simulink model "Battery_droop_control_4"  (R2022a)
settings: Solver=ode23tb  StartTime=0.0  StopTime=1  RelTol=1e-3  EnableMultiTasking=on
values from neighbouring files (symbols this model uses):
  R_power_mode_load_change = zeros(1, length(load_percent_list))    [Battery_charge_discharge_FSBB_param_init.m]
  R_voltage_mode_load_change = zeros(1, length(load_percent_list))    [Battery_charge_discharge_FSBB_param_init.m]
  time_step = 1 / wave_freq    (= 2.22222222222e-05)    [Battery_charge_discharge_FSBB_param_init.m]
undefined symbols (not defined in the file or in its folder): Ion, Lithium
libraries: spsSeriesRLCBranchLib x27, spsTriangleGeneratorLib x16, slpidlib x14, spsCurrentMeasurementLib x9, spsIGBTDiodeLib x8, spsIdealSwitchLib x8, spsVoltageMeasurementLib x8, simulink x4, spsBatteryLib x3, spsControlledVoltageSourceLib x3, eeGeneralControl x2, spspowerguiLib x1
(part 2 of 4)

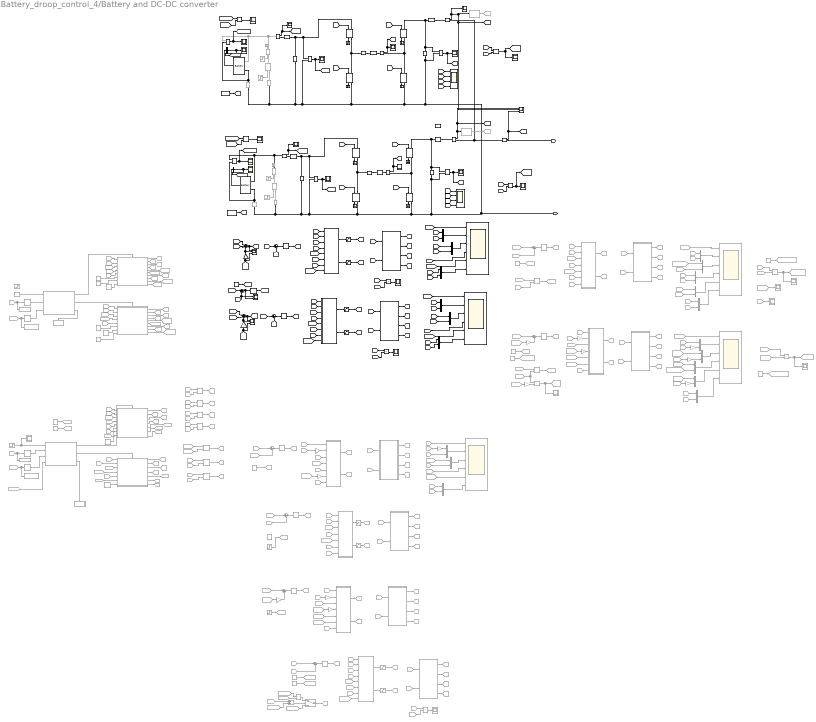
== system Battery_droop_control_4/Battery and DC-DC converter ==
  note: Discharge in Constant Power Mode : realize by constant current
  note: Be charged in constant Current Mode
  note: Discharge in constant Current Mode
  note: Discharge in constant Voltage Mode
  note: FSBB Passivity Based Control
      | control algorithm ref: https://www.youtube.com/watch?v=5YT7cERlMrg
      | 1. Modify the topology corresponding to Gosspower hardware.
      | 1.1 add additional capacities in both input and output side
      | 1.2 add additional 2.2e-6H inductor in both input and output side to mitigate the fluctuation in constant current mode.
      | 2. Realize the constant current/voltage/Power mode in charge/discharge mode.
      |
      | Author LokiXun rongji.xun@gmail.com
  note: Be Charged in constant Voltage Mode
  note: Be Charged in Constant Power Mode : realize by constant current
  note: Constant Current/Power Transition Point
  note: Charge Mode Transition
  note: Discharge Mode Transition
  note: Discharge in Constant Current Mode using Voltage control
  note: Charge Mode
  note: Discharge Mode
  note: I_imax = 31.25A; Ubus_min = 95.5V; Ubus_ref = 96V;
  note: I_imax = 31.25A; Ubus_min = 95.5V; Ubus_ref = 96V;
  note: 和开关频率同步
  note: Discharge in constant Voltage Mode
  note: 和开关频率同步
  "85 volts, 100 Ah LithiumIon battery " : spsBatteryLib/Battery  BatType=Lithium-Ion  ShowTempParam=off  ThermalPreset=no  ShowAgeParam=off  NomV=85  NomQ=100  SOC=20  Batt_Tr=30  PresetModel=off  MaxQ=107.6923  MinV=83.2  FullV=115.2  Dis_rate=43.4783  R=0.08  Normal_OP=96.1538  expZone=[92.2034, 20]  current=[6.5 13 32.5]  Units=Time  Tci=20  NomT=20  T2=-30  MaxQ2=4.8  FullV2=7.1  Normal_OP2=5.655  expZone2="[6.58           1]"  Rca=0.6  ti=2000  Dp=0  Neq0=0  Tsim=1e6  Ta1=25  Qeol=5.4*0.9  Reol=0.013333*1.2  Char_age=[2.3478, 3]  Dis_age=[2.3478, 10]  N1=1500  N2=10500  N3=1000  N4=1400  Ta2=45  N5=950
  "85 volts, 100 Ah LithiumIon battery 2" : spsBatteryLib/Battery  BatType=Lithium-Ion  ShowTempParam=off  ThermalPreset=no  ShowAgeParam=off  NomV=85  NomQ=100  SOC=20  Batt_Tr=30  PresetModel=off  MaxQ=107.6923  MinV=83.2  FullV=115.2  Dis_rate=43.4783  R=0.08  Normal_OP=96.1538  expZone=[92.2034, 20]  current=[6.5 13 32.5]  Units=Time  Tci=20  NomT=20  T2=-30  MaxQ2=4.8  FullV2=7.1  Normal_OP2=5.655  expZone2="[6.58           1]"  Rca=0.6  ti=2000  Dp=0  Neq0=0  Tsim=1e6  Ta1=25  Qeol=5.4*0.9  Reol=0.013333*1.2  Char_age=[2.3478, 3]  Dis_age=[2.3478, 10]  N1=1500  N2=10500  N3=1000  N4=1400  Ta2=45  N5=950
  ActualPower1 : Scope  Commented=on
  ActualPower2 : Scope  Commented=on
  Battery Load : Scope
  Battery Load2 : Scope
  BatteryCurrent1 : Scope  Commented=on
  Bus Selector : BusSelector  OutputSignals=SOC (%)
  Bus Selector2 : BusSelector  OutputSignals=SOC (%)
  BusPower : Scope  Commented=on
  C1 : spsSeriesRLCBranchLib/Series RLC Branch  LConnTagsString=__new0  RConnTagsString=__new0  BranchType=C  Resistance=0.01  Inductance=1e-3  SetiL0=off  InitialCurrent=0  Capacitance=1440e-6  Setx0=on  InitialVoltage=90  Measurements=None
  C2 : spsSeriesRLCBranchLib/Series RLC Branch  LConnTagsString=__new0  RConnTagsString=__new0  BranchType=C  Resistance=5  Inductance=1e-3  SetiL0=off  InitialCurrent=0  Capacitance=2440e-6  Setx0=on  InitialVoltage=90  Measurements=None
  C5 : spsSeriesRLCBranchLib/Series RLC Branch  LConnTagsString=__new0  RConnTagsString=__new0  BranchType=C  Resistance=0.01  Inductance=1e-3  SetiL0=off  InitialCurrent=0  Capacitance=1440e-6  Setx0=on  InitialVoltage=90  Measurements=None
  C6 : spsSeriesRLCBranchLib/Series RLC Branch  LConnTagsString=__new0  RConnTagsString=__new0  BranchType=C  Resistance=5  Inductance=1e-3  SetiL0=off  InitialCurrent=0  Capacitance=2440e-6  Setx0=on  InitialVoltage=90  Measurements=None
  Charge : Scope  Commented=on  NumInputPorts=6
  Charge Mixed CurrentPower : Subsystem  Commented=on  TreatAsAtomicUnit=on
  Charge Mixed CurrentPower1 : Subsystem  Commented=on  TreatAsAtomicUnit=on
  Charge/Discharge Mode2 : Constant  Commented=on  SampleTime=0
  Charge0 /Discharge1 Mode : Step  Commented=on  Time=0.5  Before=1  SampleTime=1
  Charge0 /Discharge1 Mode1 : Step  Commented=on  Time=0.3  Before=1  After=0  SampleTime=0
  Constant1 : Constant  Value=time_step
  Constant{5,7,9..10} (4 alike) : Constant  Commented=on  Value=3000
  Constant11 : Constant  Commented=on  Value=96
  Constant12 : Constant  Commented=on  Value=101
  Constant13 : Constant  Value=96
  Constant14 : Constant  Commented=on  Value=103.5
  Constant16 : Constant  Commented=on  Value=101
  Constant17 : Constant  Value=time_step
  Constant19 : Constant  Commented=on  Value=96
  Constant2 : Constant  Commented=on  Value=30
  Constant20 : Constant  Commented=on  Value=91
  Constant3 : Constant  Commented=on  Value=26
  Constant4 : Constant  Commented=on  Value=29
  Constant6 : Constant  Commented=on  Value=29
  Constant8 : Constant  Commented=on  Value=30
  Controlled Voltage Source : spsControlledVoltageSourceLib/Controlled Voltage Source  Commented=on  Initialize=on  Source_Type=DC  Amplitude=96  Phase=0  Frequency=0  Measurements=None
  Controlled Voltage Source2 : spsControlledVoltageSourceLib/Controlled Voltage Source  Commented=on  Initialize=on  Source_Type=DC  Amplitude=96  Phase=0  Frequency=0  Measurements=None
  Current 1 : spsCurrentMeasurementLib/Current Measurement  PhasorSimulation=off  OutputType=Complex  PSBequivalent=0
  Current 2 : spsCurrentMeasurementLib/Current Measurement  PhasorSimulation=off  OutputType=Complex  PSBequivalent=0
  Current Measurement : spsCurrentMeasurementLib/Current Measurement  PhasorSimulation=off  OutputType=Complex  PSBequivalent=0
  Current Measurement2 : spsCurrentMeasurementLib/Current Measurement  PhasorSimulation=off  OutputType=Complex  PSBequivalent=0
  Current total : spsCurrentMeasurementLib/Current Measurement  PhasorSimulation=off  OutputType=Complex  PSBequivalent=0
  DM_inductor1 : spsSeriesRLCBranchLib/Series RLC Branch  LConnTagsString=__new0  RConnTagsString=__new0  BranchType=L  Resistance=1.0  Inductance=2.2e-6  SetiL0=off  InitialCurrent=0  Capacitance=1.0  Setx0=off  InitialVoltage=0  Measurements=None
  DM_inductor2 : spsSeriesRLCBranchLib/Series RLC Branch  LConnTagsString=__new0  RConnTagsString=__new0  BranchType=L  Resistance=1.0  Inductance=2.5e-6  SetiL0=off  InitialCurrent=0  Capacitance=1.0  Setx0=off  InitialVoltage=0  Measurements=None
  DM_inductor3 : spsSeriesRLCBranchLib/Series RLC Branch  LConnTagsString=__new0  RConnTagsString=__new0  BranchType=L  Resistance=1.0  Inductance=2.2e-6  SetiL0=off  InitialCurrent=0  Capacitance=1.0  Setx0=off  InitialVoltage=0  Measurements=None
  DM_inductor5 : spsSeriesRLCBranchLib/Series RLC Branch  LConnTagsString=__new0  RConnTagsString=__new0  BranchType=L  Resistance=1.0  Inductance=2.2e-6  SetiL0=off  InitialCurrent=0  Capacitance=1.0  Setx0=off  InitialVoltage=0  Measurements=None
  DM_inductor6 : spsSeriesRLCBranchLib/Series RLC Branch  LConnTagsString=__new0  RConnTagsString=__new0  BranchType=L  Resistance=1.0  Inductance=2.5e-6  SetiL0=off  InitialCurrent=0  Capacitance=1.0  Setx0=off  InitialVoltage=0  Measurements=None
  Discharge : Scope  Commented=on  NumInputPorts=6
  Discharge Const Voltage : Subsystem  Commented=on  TreatAsAtomicUnit=on
  Discharge Mixed CurrentPower : Subsystem  Commented=on  TreatAsAtomicUnit=on
  Discharge+V : Scope  NumInputPorts=6
  Discharge+V1 : Scope  NumInputPorts=6
  Divide : Product  Commented=on  Inputs=*/
  Divide1 : Product  Commented=on  Inputs=*/
  Divide{2..3,6..7} (4 alike) : Product  Inputs=*/
  DoNothing1 : Subsystem  Commented=on  TreatAsAtomicUnit=on
  DoNothing2 : Subsystem  Commented=on  TreatAsAtomicUnit=on
  From{45,70,75,87,100,147,150,153} (8 alike) : From  Commented=on  GotoTag=VC_ref
  From{37..38,57..58,72,101,110,172,174,177,202} (11 alike) : From  Commented=on  GotoTag=i_out_ref
  From102 : From  Commented=on  GotoTag=Battery_SOC
  From{103,187..188,196} (4 alike) : From  Commented=on  GotoTag=Power_ref
  From{33,59..60,71,77,83,94,104,108,122,136,140,146,155,169,180,203,242} (18 alike) : From  Commented=on  GotoTag=V_battery
  From{34,41,74,91,95,106..107,121,178,197..198,243} (12 alike) : From  Commented=on  GotoTag=i_battery
  From109 : From  Commented=on  GotoTag=u2_D
  From111 : From  Commented=on  GotoTag=Power_battery
  From{86,97,112,183} (4 alike) : From  Commented=on  GotoTag=V_dc
  From{36,56,79,84,113,158,171,181,201} (9 alike) : From  Commented=on  GotoTag=iL_ref
  From{24,30,32,68,85,114,125,139,144,152,168,182,190} (13 alike) : From  Commented=on  GotoTag=iL
  From115 : From  Commented=on  GotoTag=S1_D
  From116 : From  Commented=on  GotoTag=S2_D
  From118 : From  Commented=on  GotoTag=S3_D
  From119 : From  Commented=on  GotoTag=S4_D
  From120 : From  Commented=on  GotoTag=iL_ref_D
  From{35,54,66,78,123,137,142,157,170,200} (10 alike) : From  Commented=on  GotoTag=Ts
  From{52..53,67,69,76,88,98,124,138,143,145,154,189,191,199} (15 alike) : From  Commented=on  GotoTag=V_bus
  From126 : From  Commented=on  GotoTag=S1_C
  From127 : From  Commented=on  GotoTag=S2_C
  From128 : From  Commented=on  GotoTag=S3_C
  From129 : From  Commented=on  GotoTag=S4_C
  From130 : From  Commented=on  GotoTag=iL_ref_C
  From132 : From  Commented=on  GotoTag=u1_C
  From133 : From  Commented=on  GotoTag=u2_C
  From{31,46,55,65,92,141,159,192..193} (9 alike) : From  Commented=on  GotoTag=i_out
  From156 : From  Commented=on  GotoTag=Bus_load
  From{39,49,61,64,80,89,173,185,194} (9 alike) : From  Commented=on  GotoTag=u1
  From{40,50,62,81,90,93,175,186,195} (9 alike) : From  Commented=on  GotoTag=u2
  From179 : From  Commented=on  GotoTag=Power_bus
  From184 : From  Commented=on  GotoTag=i_dc
  From244 : From  Commented=on  GotoTag=V_charge_PowerMode
  From44 : From  Commented=on  GotoTag=i_out_max_ref
  From47 : From  Commented=on  GotoTag=V_out_initial
  From48 : From  Commented=on  GotoTag=i_out_max_ref
  From51 : From  Commented=on  GotoTag=Bus_load
  From63 : From  Commented=on  GotoTag=i_dc
  From73 : From  Commented=on  GotoTag=u1_D
  From82 : From  Commented=on  GotoTag=i_dc
  From99 : From  Commented=on  GotoTag=Bus_load
  Gain{,2..3,6..8,10..12,14..17} (13 alike) : Gain  Commented=on  Gain=-1
  Goto100 : Goto  Commented=on  GotoTag=V_power_starup
  Goto{6,15,17,61,81,88,101} (7 alike) : Goto  Commented=on  GotoTag=u1
  Goto{7,18,25,62,89,102,119} (7 alike) : Goto  Commented=on  GotoTag=u2
  Goto{23,31,40,59,77,94,103} (7 alike) : Goto  Commented=on  GotoTag=S1
  Goto{24,32,41,57,78,95,104} (7 alike) : Goto  Commented=on  GotoTag=S3
  Goto105 : Goto  Commented=on  GotoTag=S4_D
  Goto107 : Goto  Commented=on  GotoTag=iL_ref_C
  Goto108 : Goto  Commented=on  GotoTag=u1_C
  Goto109 : Goto  Commented=on  GotoTag=u2_C
  Goto111 : Goto  Commented=on  GotoTag=S2_C
  Goto112 : Goto  Commented=on  GotoTag=S3_C
  Goto113 : Goto  Commented=on  GotoTag=S4_C
  Goto114 : Goto  Commented=on  GotoTag=S1_C
  Goto117 : Goto  Commented=on  GotoTag=VC_ref
  Goto120 : Goto  Commented=on  GotoTag=V_out_initial
  Goto126 : Goto  Commented=on  GotoTag=V_discharge_PowerMode
  Goto131 : Goto  Commented=on  GotoTag=i_dc
  Goto138 : Goto  Commented=on  GotoTag=i_dc2
  Goto144 : Goto  Commented=on  GotoTag=Power_battery
  Goto145 : Goto  Commented=on  GotoTag=V_charge_PowerMode
  Goto{19,26,45..46,96} (5 alike) : Goto  Commented=on  GotoTag=i_out_ref
  Goto{20,27,36,39,60,75,91} (7 alike) : Goto  Commented=on  GotoTag=iL_ref
  Goto{21,28..29,34,42,58,92} (7 alike) : Goto  Commented=on  GotoTag=S4
  Goto{22,30,33,35,43,56,93} (7 alike) : Goto  Commented=on  GotoTag=S2
  Goto37 : Goto  Commented=on  GotoTag=VC_ref
  Goto38 : Goto  Commented=on  GotoTag=Power_ref
  Goto47 : Goto  Commented=on  GotoTag=S1_D
  Goto48 : Goto  Commented=on  GotoTag=iL_ref_D
  Goto49 : Goto  Commented=on  GotoTag=u1_D
  Goto50 : Goto  Commented=on  GotoTag=u2_D
  Goto51 : Goto  Commented=on  GotoTag=i_out_ref_D
  Goto52 : Goto  Commented=on  GotoTag=S2_D
  Goto53 : Goto  Commented=on  GotoTag=S3_D
  Goto54 : Goto  Commented=on  GotoTag=S4_D
  Goto55 : Goto  Commented=on  GotoTag=Power_ref_D
  Goto65 : Goto  Commented=on  GotoTag=iL_ref_C
  Goto66 : Goto  Commented=on  GotoTag=u1_C
  Goto67 : Goto  Commented=on  GotoTag=u2_C
  Goto68 : Goto  Commented=on  GotoTag=i_out_ref_C
  Goto69 : Goto  Commented=on  GotoTag=S2_C
  Goto70 : Goto  Commented=on  GotoTag=S3_C
  Goto71 : Goto  Commented=on  GotoTag=S4_C
  Goto72 : Goto  Commented=on  GotoTag=S1_C
  Goto73 : Goto  Commented=on  GotoTag=Power_ref_C
  Goto74 : Goto  Commented=on  GotoTag=iL_PD_out
  Goto76 : Goto  Commented=on  GotoTag=VC_ref
  Goto80 : Goto  Commented=on  GotoTag=i_out_max_ref
  Goto82 : Goto  Commented=on  GotoTag=S1_D
  Goto83 : Goto  Commented=on  GotoTag=iL_ref_D
  Goto84 : Goto  Commented=on  GotoTag=u1_D
  Goto85 : Goto  Commented=on  GotoTag=u2_D
  Goto87 : Goto  Commented=on  GotoTag=S2_D
  Goto90 : Goto  Commented=on  GotoTag=Power_ref
  Goto97 : Goto  Commented=on  GotoTag=Power_bus
  Goto98 : Goto  Commented=on  GotoTag=S3_D
  Goto99 : Goto  Commented=on  GotoTag=Power_out
  IGBT/Diode{1..4,9..12} (8 alike) : spsIGBTDiodeLib/IGBT//Diode  Ron=1e-3  Rs=1e5  Cs=inf  Measurements=on
  IL2 : spsCurrentMeasurementLib/Current Measurement  PhasorSimulation=off  OutputType=Complex  PSBequivalent=0
  IL6 : spsCurrentMeasurementLib/Current Measurement  PhasorSimulation=off  OutputType=Complex  PSBequivalent=0
  Ideal Switch2 : spsIdealSwitchLib/Ideal Switch  Commented=on  Ron=0.001  Lon=0  IC=0  Rs=1e5  Cs=inf  Measurements=on
  Ideal Switch3 : spsIdealSwitchLib/Ideal Switch  Commented=on  Ron=0.001  Lon=0  IC=0  Rs=1e5  Cs=inf  Measurements=on
  If1 : If  Commented=on  NumInputs=4  IfExpression="u1 == 1  & u4 > 10"  ElseIfExpressions=u1 == 0 & u4 < 95
  If2 : If  Commented=on  NumInputs=3  IfExpression=u1 == 1 & (u2>=87.9 & u2 <= 119)  ElseIfExpressions=u1 == 0 & (u3>=85.5 & u3 <= 116.15)
  InductorCurrent : Scope
  InductorCurrent2 : Scope
  Low-Pass Filter (Discrete or Continuous) : eeGeneralControl/Low-Pass Filter (Discrete or Continuous)  Commented=on  K=1  T=1  B=inf  A=-inf  init_option=Inherited from block input  x0=0  Ts=-1
  Low-Pass Filter (Discrete or Continuous)1 : eeGeneralControl/Low-Pass Filter (Discrete or Continuous)  Commented=on  K=1  T=1  B=inf  A=-inf  init_option=Inherited from block input  x0=0  Ts=-1
  MATLAB Function : MATLAB Function  TreatAsAtomicUnit=on
  MATLAB Function1 : MATLAB Function  Commented=on  TreatAsAtomicUnit=on
  MATLAB Function2 : MATLAB Function  Commented=on  TreatAsAtomicUnit=on
  MATLAB Function3 : MATLAB Function  Commented=on  TreatAsAtomicUnit=on
  MATLAB Function4 : MATLAB Function  TreatAsAtomicUnit=on
  MATLAB Function5 : MATLAB Function  Commented=on  TreatAsAtomicUnit=on
  MATLAB Function6 : MATLAB Function  Commented=on  TreatAsAtomicUnit=on
  MATLAB Function7 : MATLAB Function  Commented=on  TreatAsAtomicUnit=on
  Minus : Sum  Commented=on  Inputs=+-
  Modulation : Subsystem
  Modulation1 : Subsystem  Commented=on
  Modulation2 : Subsystem  Commented=on
  Modulation3 : Subsystem  Commented=on
  Modulation4 : Subsystem  Commented=on
  Modulation5 : Subsystem  Commented=on
  Modulation6 : Subsystem  Commented=on
  Modulation7 : Subsystem
  Mux{,1..5} (6 alike) : Mux  Inputs=2
  Mux{9..21} (13 alike) : Mux  Commented=on  Inputs=2
  Outside Load : Scope
  Outside Load2 : Scope
  PID Controller : slpidlib/PID Controller  Controller=PI  Form=Parallel  TimeDomain=Continuous-time  UseExternalTs=off  SampleTime=-1  IntegratorMethod=Forward Euler  FilterMethod=Forward Euler  ControllerParametersSource=internal  P=1.8  I=10000  UseKiTs=off  D=0  N=100  UseFilter=on  TunerSelectOption=Transfer Function Based (PID Tuner App)  InitialConditionSource=internal  InitialConditionForIntegrator=0  InitialConditionForFilter=0  DifferentiatorICPrevScaledInput=0  ExternalReset=none  TrackingMode=off  Kt=1  LimitOutput=off  SatLimitsSource=internal  UpperSaturationLimit=inf  LowerSaturationLimit=-inf  LinearizeAsGain=on  AntiWindupMode=none  Kb=1  POutMin=[]  POutMax=[]  IOutMin=[]  IOutMax=[]  DOutMin=[]  DOutMax=[]  NOutMin=[]  NOutMax=[]  SumOutMin=[]  SumOutMax=[]  SaturationOutMin=[]  SaturationOutMax=[]  PParamMin=[]  PParamMax=[]  IParamMin=[]  IParamMax=[]  DParamMin=[]  DParamMax=[]  NParamMin=[]  NParamMax=[]  KbParamMin=[]  KbParamMax=[]  KtParamMin=[]  KtParamMax=[]  KbOutMin=[]  KbOutMax=[]  KtOutMin=[]  KtOutMax=[]  IntegratorOutMin=[]  IntegratorOutMax=[]  FilterOutMin=[]  FilterOutMax=[]  SumI1OutMin=[]  SumI1OutMax=[]  SumI2OutMin=[]  SumI2OutMax=[]  SumI3OutMin=[]  SumI3OutMax=[]  SumI4OutMin=[]  SumI4OutMax=[]  SumDOutMin=[]  SumDOutMax=[]  DifferentiatorOutMin=[]  DifferentiatorOutMax=[]  FilterDiffOutCoefMin=[]  FilterDiffOutCoefMax=[]  ReciprocalOutMin=[]  ReciprocalOutMax=[]  SumDenOutMin=[]  SumDenOutMax=[]  SumNumOutMin=[]  SumNumOutMax=[]  DivideOutMin=[]  DivideOutMax=[]  UdiffTsProdOutMin=[]  UdiffTsProdOutMax=[]  NTsProdOutMin=[]  NTsProdOutMax=[]  UintegralTsProdOutMin=[]  UintegralTsProdOutMax=[]  UngainTsProdOutMin=[]  UngainTsProdOutMax=[]  IntegratorContinuousStateAttributes=''  IntegratorStateMustResolveToSignalObject=off  IntegratorRTWStateStorageClass=Auto  FilterContinuousStateAttributes=''  FilterStateMustResolveToSignalObject=off  FilterRTWStateStorageClass=Auto  ParallelPVariant=InternalParameters  IdealPVariant=Disabled  IVariant=InternalParameters  DVariant=Disabled  IntegratorVariant=Continuous  SatVariant=Disabled  AWVariant=Passthrough  PCopyVariant=Disabled  TRVariant=Disabled  FdbkBlocksVariant=Forward  IdealPFdbkVariant=Disabled  SatFdbkVariant=Disabled  DerivativeFilterVariant=Disabled  NVariant=Disabled  NCopyVariant=Disabled_SignalSpec  FilterICVariant=Disabled  IntegratorICVariant=InternalICs  ExternalResetVariant=Disabled  TRSumVariant=Passthrough  SumFdbkVariant=Disabled  SumVariant=Sum_PI  TsampFilterVariant=InternalTs  TsampNgainVariant=Passthrough  TsampIntegralVariant=Passthrough  ExternalSaturationOutDataTypeStr=Inherit: Same as second input  aMode=0
  PID Controller1 : slpidlib/PID Controller  Commented=on  Controller=PI  Form=Parallel  TimeDomain=Continuous-time  UseExternalTs=off  SampleTime=-1  IntegratorMethod=Forward Euler  FilterMethod=Forward Euler  ControllerParametersSource=internal  P=6.7500  I=8.1000e+03 * 2  UseKiTs=on  D=0  N=100  UseFilter=on  TunerSelectOption=Transfer Function Based (PID Tuner App)  InitialConditionSource=internal  InitialConditionForIntegrator=0  InitialConditionForFilter=0  DifferentiatorICPrevScaledInput=0  ExternalReset=none  TrackingMode=off  Kt=1  LimitOutput=on  SatLimitsSource=internal  UpperSaturationLimit=50  LowerSaturationLimit=-10  LinearizeAsGain=on  AntiWindupMode=none  Kb=1  POutMin=[]  POutMax=[]  IOutMin=[]  IOutMax=[]  DOutMin=[]  DOutMax=[]  NOutMin=[]  NOutMax=[]  SumOutMin=[]  SumOutMax=[]  SaturationOutMin=[]  SaturationOutMax=[]  PParamMin=[]  PParamMax=[]  IParamMin=[]  IParamMax=[]  DParamMin=[]  DParamMax=[]  NParamMin=[]  NParamMax=[]  KbParamMin=[]  KbParamMax=[]  KtParamMin=[]  KtParamMax=[]  KbOutMin=[]  KbOutMax=[]  KtOutMin=[]  KtOutMax=[]  IntegratorOutMin=[]  IntegratorOutMax=[]  FilterOutMin=[]  FilterOutMax=[]  SumI1OutMin=[]  SumI1OutMax=[]  SumI2OutMin=[]  SumI2OutMax=[]  SumI3OutMin=[]  SumI3OutMax=[]  SumI4OutMin=[]  SumI4OutMax=[]  SumDOutMin=[]  SumDOutMax=[]  DifferentiatorOutMin=[]  DifferentiatorOutMax=[]  FilterDiffOutCoefMin=[]  FilterDiffOutCoefMax=[]  ReciprocalOutMin=[]  ReciprocalOutMax=[]  SumDenOutMin=[]  SumDenOutMax=[]  SumNumOutMin=[]  SumNumOutMax=[]  DivideOutMin=[]  DivideOutMax=[]  UdiffTsProdOutMin=[]  UdiffTsProdOutMax=[]  NTsProdOutMin=[]  NTsProdOutMax=[]  UintegralTsProdOutMin=[]  UintegralTsProdOutMax=[]  UngainTsProdOutMin=[]  UngainTsProdOutMax=[]  IntegratorContinuousStateAttributes=''  IntegratorStateMustResolveToSignalObject=off  IntegratorRTWStateStorageClass=Auto  FilterContinuousStateAttributes=''  FilterStateMustResolveToSignalObject=off  FilterRTWStateStorageClass=Auto  ParallelPVariant=InternalParameters  IdealPVariant=Disabled  IVariant=InternalParameters  DVariant=Disabled  IntegratorVariant=Continuous  SatVariant=Enabled  AWVariant=Passthrough  PCopyVariant=Disabled  TRVariant=Disabled  FdbkBlocksVariant=Forward  IdealPFdbkVariant=Disabled  SatFdbkVariant=Disabled  DerivativeFilterVariant=Disabled  NVariant=Disabled  NCopyVariant=Disabled_SignalSpec  FilterICVariant=Disabled  IntegratorICVariant=InternalICs  ExternalResetVariant=Disabled  TRSumVariant=Passthrough  SumFdbkVariant=Disabled  SumVariant=Sum_PI  TsampFilterVariant=InternalTs  TsampNgainVariant=Passthrough  TsampIntegralVariant=Passthrough  ExternalSaturationOutDataTypeStr=Inherit: Same as second input  aMode=0
  PID Controller2 : slpidlib/PID Controller  Controller=PI  Form=Parallel  TimeDomain=Continuous-time  UseExternalTs=off  SampleTime=-1  IntegratorMethod=Forward Euler  FilterMethod=Forward Euler  ControllerParametersSource=internal  P=45 * 2  I=1.3361e+05 /25  UseKiTs=on  D=0  N=100  UseFilter=on  TunerSelectOption=Frequency Response Based  InitialConditionSource=internal  InitialConditionForIntegrator=0  InitialConditionForFilter=0  DifferentiatorICPrevScaledInput=0  ExternalReset=none  TrackingMode=off  Kt=1  LimitOutput=on  SatLimitsSource=internal  UpperSaturationLimit=50  LowerSaturationLimit=-10  LinearizeAsGain=on  AntiWindupMode=none  Kb=1  POutMin=[]  POutMax=[]  IOutMin=[]  IOutMax=[]  DOutMin=[]  DOutMax=[]  NOutMin=[]  NOutMax=[]  SumOutMin=[]  SumOutMax=[]  SaturationOutMin=[]  SaturationOutMax=[]  PParamMin=[]  PParamMax=[]  IParamMin=[]  IParamMax=[]  DParamMin=[]  DParamMax=[]  NParamMin=[]  NParamMax=[]  KbParamMin=[]  KbParamMax=[]  KtParamMin=[]  KtParamMax=[]  KbOutMin=[]  KbOutMax=[]  KtOutMin=[]  KtOutMax=[]  IntegratorOutMin=[]  IntegratorOutMax=[]  FilterOutMin=[]  FilterOutMax=[]  SumI1OutMin=[]  SumI1OutMax=[]  SumI2OutMin=[]  SumI2OutMax=[]  SumI3OutMin=[]  SumI3OutMax=[]  SumI4OutMin=[]  SumI4OutMax=[]  SumDOutMin=[]  SumDOutMax=[]  DifferentiatorOutMin=[]  DifferentiatorOutMax=[]  FilterDiffOutCoefMin=[]  FilterDiffOutCoefMax=[]  ReciprocalOutMin=[]  ReciprocalOutMax=[]  SumDenOutMin=[]  SumDenOutMax=[]  SumNumOutMin=[]  SumNumOutMax=[]  DivideOutMin=[]  DivideOutMax=[]  UdiffTsProdOutMin=[]  UdiffTsProdOutMax=[]  NTsProdOutMin=[]  NTsProdOutMax=[]  UintegralTsProdOutMin=[]  UintegralTsProdOutMax=[]  UngainTsProdOutMin=[]  UngainTsProdOutMax=[]  IntegratorContinuousStateAttributes=''  IntegratorStateMustResolveToSignalObject=off  IntegratorRTWStateStorageClass=Auto  FilterContinuousStateAttributes=''  FilterStateMustResolveToSignalObject=off  FilterRTWStateStorageClass=Auto  ParallelPVariant=InternalParameters  IdealPVariant=Disabled  IVariant=InternalParameters  DVariant=Disabled  IntegratorVariant=Continuous  SatVariant=Enabled  AWVariant=Passthrough  PCopyVariant=Disabled  TRVariant=Disabled  FdbkBlocksVariant=Forward  IdealPFdbkVariant=Disabled  SatFdbkVariant=Disabled  DerivativeFilterVariant=Disabled  NVariant=Disabled  NCopyVariant=Disabled_SignalSpec  FilterICVariant=Disabled  IntegratorICVariant=InternalICs  ExternalResetVariant=Disabled  TRSumVariant=Passthrough  SumFdbkVariant=Disabled  SumVariant=Sum_PI  TsampFilterVariant=InternalTs  TsampNgainVariant=Passthrough  TsampIntegralVariant=Passthrough  ExternalSaturationOutDataTypeStr=Inherit: Same as second input  aMode=0
  PID Controller3 : slpidlib/PID Controller  Commented=on  Controller=PI  Form=Parallel  TimeDomain=Continuous-time  UseExternalTs=off  SampleTime=-1  IntegratorMethod=Forward Euler  FilterMethod=Forward Euler  ControllerParametersSource=internal  P=6.7500  I=8.1000e+03 * 2  UseKiTs=on  D=0  N=100  UseFilter=on  TunerSelectOption=Transfer Function Based (PID Tuner App)  InitialConditionSource=internal  InitialConditionForIntegrator=0  InitialConditionForFilter=0  DifferentiatorICPrevScaledInput=0  ExternalReset=none  TrackingMode=off  Kt=1  LimitOutput=on  SatLimitsSource=internal  UpperSaturationLimit=50  LowerSaturationLimit=-10  LinearizeAsGain=on  AntiWindupMode=none  Kb=1  POutMin=[]  POutMax=[]  IOutMin=[]  IOutMax=[]  DOutMin=[]  DOutMax=[]  NOutMin=[]  NOutMax=[]  SumOutMin=[]  SumOutMax=[]  SaturationOutMin=[]  SaturationOutMax=[]  PParamMin=[]  PParamMax=[]  IParamMin=[]  IParamMax=[]  DParamMin=[]  DParamMax=[]  NParamMin=[]  NParamMax=[]  KbParamMin=[]  KbParamMax=[]  KtParamMin=[]  KtParamMax=[]  KbOutMin=[]  KbOutMax=[]  KtOutMin=[]  KtOutMax=[]  IntegratorOutMin=[]  IntegratorOutMax=[]  FilterOutMin=[]  FilterOutMax=[]  SumI1OutMin=[]  SumI1OutMax=[]  SumI2OutMin=[]  SumI2OutMax=[]  SumI3OutMin=[]  SumI3OutMax=[]  SumI4OutMin=[]  SumI4OutMax=[]  SumDOutMin=[]  SumDOutMax=[]  DifferentiatorOutMin=[]  DifferentiatorOutMax=[]  FilterDiffOutCoefMin=[]  FilterDiffOutCoefMax=[]  ReciprocalOutMin=[]  ReciprocalOutMax=[]  SumDenOutMin=[]  SumDenOutMax=[]  SumNumOutMin=[]  SumNumOutMax=[]  DivideOutMin=[]  DivideOutMax=[]  UdiffTsProdOutMin=[]  UdiffTsProdOutMax=[]  NTsProdOutMin=[]  NTsProdOutMax=[]  UintegralTsProdOutMin=[]  UintegralTsProdOutMax=[]  UngainTsProdOutMin=[]  UngainTsProdOutMax=[]  IntegratorContinuousStateAttributes=''  IntegratorStateMustResolveToSignalObject=off  IntegratorRTWStateStorageClass=Auto  FilterContinuousStateAttributes=''  FilterStateMustResolveToSignalObject=off  FilterRTWStateStorageClass=Auto  ParallelPVariant=InternalParameters  IdealPVariant=Disabled  IVariant=InternalParameters  DVariant=Disabled  IntegratorVariant=Continuous  SatVariant=Enabled  AWVariant=Passthrough  PCopyVariant=Disabled  TRVariant=Disabled  FdbkBlocksVariant=Forward  IdealPFdbkVariant=Disabled  SatFdbkVariant=Disabled  DerivativeFilterVariant=Disabled  NVariant=Disabled  NCopyVariant=Disabled_SignalSpec  FilterICVariant=Disabled  IntegratorICVariant=InternalICs  ExternalResetVariant=Disabled  TRSumVariant=Passthrough  SumFdbkVariant=Disabled  SumVariant=Sum_PI  TsampFilterVariant=InternalTs  TsampNgainVariant=Passthrough  TsampIntegralVariant=Passthrough  ExternalSaturationOutDataTypeStr=Inherit: Same as second input  aMode=0
  PID Controller4 : slpidlib/PID Controller  Commented=on  Controller=PI  Form=Parallel  TimeDomain=Continuous-time  UseExternalTs=off  SampleTime=-1  IntegratorMethod=Forward Euler  FilterMethod=Forward Euler  ControllerParametersSource=internal  P=15  I=1000  UseKiTs=on  D=0  N=100  UseFilter=on  TunerSelectOption=Transfer Function Based (PID Tuner App)  InitialConditionSource=internal  InitialConditionForIntegrator=0  InitialConditionForFilter=0  DifferentiatorICPrevScaledInput=0  ExternalReset=none  TrackingMode=off  Kt=1  LimitOutput=on  SatLimitsSource=internal  UpperSaturationLimit=50  LowerSaturationLimit=-10  LinearizeAsGain=on  AntiWindupMode=none  Kb=1  POutMin=[]  POutMax=[]  IOutMin=[]  IOutMax=[]  DOutMin=[]  DOutMax=[]  NOutMin=[]  NOutMax=[]  SumOutMin=[]  SumOutMax=[]  SaturationOutMin=[]  SaturationOutMax=[]  PParamMin=[]  PParamMax=[]  IParamMin=[]  IParamMax=[]  DParamMin=[]  DParamMax=[]  NParamMin=[]  NParamMax=[]  KbParamMin=[]  KbParamMax=[]  KtParamMin=[]  KtParamMax=[]  KbOutMin=[]  KbOutMax=[]  KtOutMin=[]  KtOutMax=[]  IntegratorOutMin=[]  IntegratorOutMax=[]  FilterOutMin=[]  FilterOutMax=[]  SumI1OutMin=[]  SumI1OutMax=[]  SumI2OutMin=[]  SumI2OutMax=[]  SumI3OutMin=[]  SumI3OutMax=[]  SumI4OutMin=[]  SumI4OutMax=[]  SumDOutMin=[]  SumDOutMax=[]  DifferentiatorOutMin=[]  DifferentiatorOutMax=[]  FilterDiffOutCoefMin=[]  FilterDiffOutCoefMax=[]  ReciprocalOutMin=[]  ReciprocalOutMax=[]  SumDenOutMin=[]  SumDenOutMax=[]  SumNumOutMin=[]  SumNumOutMax=[]  DivideOutMin=[]  DivideOutMax=[]  UdiffTsProdOutMin=[]  UdiffTsProdOutMax=[]  NTsProdOutMin=[]  NTsProdOutMax=[]  UintegralTsProdOutMin=[]  UintegralTsProdOutMax=[]  UngainTsProdOutMin=[]  UngainTsProdOutMax=[]  IntegratorContinuousStateAttributes=''  IntegratorStateMustResolveToSignalObject=off  IntegratorRTWStateStorageClass=Auto  FilterContinuousStateAttributes=''  FilterStateMustResolveToSignalObject=off  FilterRTWStateStorageClass=Auto  ParallelPVariant=InternalParameters  IdealPVariant=Disabled  IVariant=InternalParameters  DVariant=Disabled  IntegratorVariant=Continuous  SatVariant=Enabled  AWVariant=Passthrough  PCopyVariant=Disabled  TRVariant=Disabled  FdbkBlocksVariant=Forward  IdealPFdbkVariant=Disabled  SatFdbkVariant=Disabled  DerivativeFilterVariant=Disabled  NVariant=Disabled  NCopyVariant=Disabled_SignalSpec  FilterICVariant=Disabled  IntegratorICVariant=InternalICs  ExternalResetVariant=Disabled  TRSumVariant=Passthrough  SumFdbkVariant=Disabled  SumVariant=Sum_PI  TsampFilterVariant=InternalTs  TsampNgainVariant=Passthrough  TsampIntegralVariant=Passthrough  ExternalSaturationOutDataTypeStr=Inherit: Same as second input  aMode=0
  PID Controller5 : slpidlib/PID Controller  Commented=on  Controller=PI  Form=Parallel  TimeDomain=Continuous-time  UseExternalTs=off  SampleTime=-1  IntegratorMethod=Forward Euler  FilterMethod=Forward Euler  ControllerParametersSource=internal  P=15  I=1000  UseKiTs=on  D=0  N=100  UseFilter=on  TunerSelectOption=Transfer Function Based (PID Tuner App)  InitialConditionSource=internal  InitialConditionForIntegrator=0  InitialConditionForFilter=0  DifferentiatorICPrevScaledInput=0  ExternalReset=none  TrackingMode=off  Kt=1  LimitOutput=on  SatLimitsSource=internal  UpperSaturationLimit=50  LowerSaturationLimit=-10  LinearizeAsGain=on  AntiWindupMode=none  Kb=1  POutMin=[]  POutMax=[]  IOutMin=[]  IOutMax=[]  DOutMin=[]  DOutMax=[]  NOutMin=[]  NOutMax=[]  SumOutMin=[]  SumOutMax=[]  SaturationOutMin=[]  SaturationOutMax=[]  PParamMin=[]  PParamMax=[]  IParamMin=[]  IParamMax=[]  DParamMin=[]  DParamMax=[]  NParamMin=[]  NParamMax=[]  KbParamMin=[]  KbParamMax=[]  KtParamMin=[]  KtParamMax=[]  KbOutMin=[]  KbOutMax=[]  KtOutMin=[]  KtOutMax=[]  IntegratorOutMin=[]  IntegratorOutMax=[]  FilterOutMin=[]  FilterOutMax=[]  SumI1OutMin=[]  SumI1OutMax=[]  SumI2OutMin=[]  SumI2OutMax=[]  SumI3OutMin=[]  SumI3OutMax=[]  SumI4OutMin=[]  SumI4OutMax=[]  SumDOutMin=[]  SumDOutMax=[]  DifferentiatorOutMin=[]  DifferentiatorOutMax=[]  FilterDiffOutCoefMin=[]  FilterDiffOutCoefMax=[]  ReciprocalOutMin=[]  ReciprocalOutMax=[]  SumDenOutMin=[]  SumDenOutMax=[]  SumNumOutMin=[]  SumNumOutMax=[]  DivideOutMin=[]  DivideOutMax=[]  UdiffTsProdOutMin=[]  UdiffTsProdOutMax=[]  NTsProdOutMin=[]  NTsProdOutMax=[]  UintegralTsProdOutMin=[]  UintegralTsProdOutMax=[]  UngainTsProdOutMin=[]  UngainTsProdOutMax=[]  IntegratorContinuousStateAttributes=''  IntegratorStateMustResolveToSignalObject=off  IntegratorRTWStateStorageClass=Auto  FilterContinuousStateAttributes=''  FilterStateMustResolveToSignalObject=off  FilterRTWStateStorageClass=Auto  ParallelPVariant=InternalParameters  IdealPVariant=Disabled  IVariant=InternalParameters  DVariant=Disabled  IntegratorVariant=Continuous  SatVariant=Enabled  AWVariant=Passthrough  PCopyVariant=Disabled  TRVariant=Disabled  FdbkBlocksVariant=Forward  IdealPFdbkVariant=Disabled  SatFdbkVariant=Disabled  DerivativeFilterVariant=Disabled  NVariant=Disabled  NCopyVariant=Disabled_SignalSpec  FilterICVariant=Disabled  IntegratorICVariant=InternalICs  ExternalResetVariant=Disabled  TRSumVariant=Passthrough  SumFdbkVariant=Disabled  SumVariant=Sum_PI  TsampFilterVariant=InternalTs  TsampNgainVariant=Passthrough  TsampIntegralVariant=Passthrough  ExternalSaturationOutDataTypeStr=Inherit: Same as second input  aMode=0
  PID Controller6 : slpidlib/PID Controller  Commented=on  Controller=PI  Form=Parallel  TimeDomain=Continuous-time  UseExternalTs=off  SampleTime=-1  IntegratorMethod=Forward Euler  FilterMethod=Forward Euler  ControllerParametersSource=internal  P=15  I=1000  UseKiTs=on  D=0  N=100  UseFilter=on  TunerSelectOption=Transfer Function Based (PID Tuner App)  InitialConditionSource=internal  InitialConditionForIntegrator=0  InitialConditionForFilter=0  DifferentiatorICPrevScaledInput=0  ExternalReset=none  TrackingMode=off  Kt=1  LimitOutput=on  SatLimitsSource=internal  UpperSaturationLimit=50  LowerSaturationLimit=-10  LinearizeAsGain=on  AntiWindupMode=none  Kb=1  POutMin=[]  POutMax=[]  IOutMin=[]  IOutMax=[]  DOutMin=[]  DOutMax=[]  NOutMin=[]  NOutMax=[]  SumOutMin=[]  SumOutMax=[]  SaturationOutMin=[]  SaturationOutMax=[]  PParamMin=[]  PParamMax=[]  IParamMin=[]  IParamMax=[]  DParamMin=[]  DParamMax=[]  NParamMin=[]  NParamMax=[]  KbParamMin=[]  KbParamMax=[]  KtParamMin=[]  KtParamMax=[]  KbOutMin=[]  KbOutMax=[]  KtOutMin=[]  KtOutMax=[]  IntegratorOutMin=[]  IntegratorOutMax=[]  FilterOutMin=[]  FilterOutMax=[]  SumI1OutMin=[]  SumI1OutMax=[]  SumI2OutMin=[]  SumI2OutMax=[]  SumI3OutMin=[]  SumI3OutMax=[]  SumI4OutMin=[]  SumI4OutMax=[]  SumDOutMin=[]  SumDOutMax=[]  DifferentiatorOutMin=[]  DifferentiatorOutMax=[]  FilterDiffOutCoefMin=[]  FilterDiffOutCoefMax=[]  ReciprocalOutMin=[]  ReciprocalOutMax=[]  SumDenOutMin=[]  SumDenOutMax=[]  SumNumOutMin=[]  SumNumOutMax=[]  DivideOutMin=[]  DivideOutMax=[]  UdiffTsProdOutMin=[]  UdiffTsProdOutMax=[]  NTsProdOutMin=[]  NTsProdOutMax=[]  UintegralTsProdOutMin=[]  UintegralTsProdOutMax=[]  UngainTsProdOutMin=[]  UngainTsProdOutMax=[]  IntegratorContinuousStateAttributes=''  IntegratorStateMustResolveToSignalObject=off  IntegratorRTWStateStorageClass=Auto  FilterContinuousStateAttributes=''  FilterStateMustResolveToSignalObject=off  FilterRTWStateStorageClass=Auto  ParallelPVariant=InternalParameters  IdealPVariant=Disabled  IVariant=InternalParameters  DVariant=Disabled  IntegratorVariant=Continuous  SatVariant=Enabled  AWVariant=Passthrough  PCopyVariant=Disabled  TRVariant=Disabled  FdbkBlocksVariant=Forward  IdealPFdbkVariant=Disabled  SatFdbkVariant=Disabled  DerivativeFilterVariant=Disabled  NVariant=Disabled  NCopyVariant=Disabled_SignalSpec  FilterICVariant=Disabled  IntegratorICVariant=InternalICs  ExternalResetVariant=Disabled  TRSumVariant=Passthrough  SumFdbkVariant=Disabled  SumVariant=Sum_PI  TsampFilterVariant=InternalTs  TsampNgainVariant=Passthrough  TsampIntegralVariant=Passthrough  ExternalSaturationOutDataTypeStr=Inherit: Same as second input  aMode=0
  PID Controller7 : slpidlib/PID Controller  Commented=on  Controller=PI  Form=Parallel  TimeDomain=Continuous-time  UseExternalTs=off  SampleTime=-1  IntegratorMethod=Forward Euler  FilterMethod=Forward Euler  ControllerParametersSource=internal  P=45 * 2  I=1.3361e+05 /25  UseKiTs=on  D=0  N=100  UseFilter=on  TunerSelectOption=Transfer Function Based (PID Tuner App)  InitialConditionSource=internal  InitialConditionForIntegrator=0  InitialConditionForFilter=0  DifferentiatorICPrevScaledInput=0  ExternalReset=none  TrackingMode=off  Kt=1  LimitOutput=on  SatLimitsSource=internal  UpperSaturationLimit=50  LowerSaturationLimit=-10  LinearizeAsGain=on  AntiWindupMode=none  Kb=1  POutMin=[]  POutMax=[]  IOutMin=[]  IOutMax=[]  DOutMin=[]  DOutMax=[]  NOutMin=[]  NOutMax=[]  SumOutMin=[]  SumOutMax=[]  SaturationOutMin=[]  SaturationOutMax=[]  PParamMin=[]  PParamMax=[]  IParamMin=[]  IParamMax=[]  DParamMin=[]  DParamMax=[]  NParamMin=[]  NParamMax=[]  KbParamMin=[]  KbParamMax=[]  KtParamMin=[]  KtParamMax=[]  KbOutMin=[]  KbOutMax=[]  KtOutMin=[]  KtOutMax=[]  IntegratorOutMin=[]  IntegratorOutMax=[]  FilterOutMin=[]  FilterOutMax=[]  SumI1OutMin=[]  SumI1OutMax=[]  SumI2OutMin=[]  SumI2OutMax=[]  SumI3OutMin=[]  SumI3OutMax=[]  SumI4OutMin=[]  SumI4OutMax=[]  SumDOutMin=[]  SumDOutMax=[]  DifferentiatorOutMin=[]  DifferentiatorOutMax=[]  FilterDiffOutCoefMin=[]  FilterDiffOutCoefMax=[]  ReciprocalOutMin=[]  ReciprocalOutMax=[]  SumDenOutMin=[]  SumDenOutMax=[]  SumNumOutMin=[]  SumNumOutMax=[]  DivideOutMin=[]  DivideOutMax=[]  UdiffTsProdOutMin=[]  UdiffTsProdOutMax=[]  NTsProdOutMin=[]  NTsProdOutMax=[]  UintegralTsProdOutMin=[]  UintegralTsProdOutMax=[]  UngainTsProdOutMin=[]  UngainTsProdOutMax=[]  IntegratorContinuousStateAttributes=''  IntegratorStateMustResolveToSignalObject=off  IntegratorRTWStateStorageClass=Auto  FilterContinuousStateAttributes=''  FilterStateMustResolveToSignalObject=off  FilterRTWStateStorageClass=Auto  ParallelPVariant=InternalParameters  IdealPVariant=Disabled  IVariant=InternalParameters  DVariant=Disabled  IntegratorVariant=Continuous  SatVariant=Enabled  AWVariant=Passthrough  PCopyVariant=Disabled  TRVariant=Disabled  FdbkBlocksVariant=Forward  IdealPFdbkVariant=Disabled  SatFdbkVariant=Disabled  DerivativeFilterVariant=Disabled  NVariant=Disabled  NCopyVariant=Disabled_SignalSpec  FilterICVariant=Disabled  IntegratorICVariant=InternalICs  ExternalResetVariant=Disabled  TRSumVariant=Passthrough  SumFdbkVariant=Disabled  SumVariant=Sum_PI  TsampFilterVariant=InternalTs  TsampNgainVariant=Passthrough  TsampIntegralVariant=Passthrough  ExternalSaturationOutDataTypeStr=Inherit: Same as second input  aMode=0
  PID Controller8 : slpidlib/PID Controller  Controller=PI  Form=Parallel  TimeDomain=Continuous-time  UseExternalTs=off  SampleTime=-1  IntegratorMethod=Forward Euler  FilterMethod=Forward Euler  ControllerParametersSource=internal  P=45 * 2  I=1.3361e+05 /25  UseKiTs=on  D=0  N=100  UseFilter=on  TunerSelectOption=Frequency Response Based  InitialConditionSource=internal  InitialConditionForIntegrator=0  InitialConditionForFilter=0  DifferentiatorICPrevScaledInput=0  ExternalReset=none  TrackingMode=off  Kt=1  LimitOutput=on  SatLimitsSource=internal  UpperSaturationLimit=50  LowerSaturationLimit=-10  LinearizeAsGain=on  AntiWindupMode=none  Kb=1  POutMin=[]  POutMax=[]  IOutMin=[]  IOutMax=[]  DOutMin=[]  DOutMax=[]  NOutMin=[]  NOutMax=[]  SumOutMin=[]  SumOutMax=[]  SaturationOutMin=[]  SaturationOutMax=[]  PParamMin=[]  PParamMax=[]  IParamMin=[]  IParamMax=[]  DParamMin=[]  DParamMax=[]  NParamMin=[]  NParamMax=[]  KbParamMin=[]  KbParamMax=[]  KtParamMin=[]  KtParamMax=[]  KbOutMin=[]  KbOutMax=[]  KtOutMin=[]  KtOutMax=[]  IntegratorOutMin=[]  IntegratorOutMax=[]  FilterOutMin=[]  FilterOutMax=[]  SumI1OutMin=[]  SumI1OutMax=[]  SumI2OutMin=[]  SumI2OutMax=[]  SumI3OutMin=[]  SumI3OutMax=[]  SumI4OutMin=[]  SumI4OutMax=[]  SumDOutMin=[]  SumDOutMax=[]  DifferentiatorOutMin=[]  DifferentiatorOutMax=[]  FilterDiffOutCoefMin=[]  FilterDiffOutCoefMax=[]  ReciprocalOutMin=[]  ReciprocalOutMax=[]  SumDenOutMin=[]  SumDenOutMax=[]  SumNumOutMin=[]  SumNumOutMax=[]  DivideOutMin=[]  DivideOutMax=[]  UdiffTsProdOutMin=[]  UdiffTsProdOutMax=[]  NTsProdOutMin=[]  NTsProdOutMax=[]  UintegralTsProdOutMin=[]  UintegralTsProdOutMax=[]  UngainTsProdOutMin=[]  UngainTsProdOutMax=[]  IntegratorContinuousStateAttributes=''  IntegratorStateMustResolveToSignalObject=off  IntegratorRTWStateStorageClass=Auto  FilterContinuousStateAttributes=''  FilterStateMustResolveToSignalObject=off  FilterRTWStateStorageClass=Auto  ParallelPVariant=InternalParameters  IdealPVariant=Disabled  IVariant=InternalParameters  DVariant=Disabled  IntegratorVariant=Continuous  SatVariant=Enabled  AWVariant=Passthrough  PCopyVariant=Disabled  TRVariant=Disabled  FdbkBlocksVariant=Forward  IdealPFdbkVariant=Disabled  SatFdbkVariant=Disabled  DerivativeFilterVariant=Disabled  NVariant=Disabled  NCopyVariant=Disabled_SignalSpec  FilterICVariant=Disabled  IntegratorICVariant=InternalICs  ExternalResetVariant=Disabled  TRSumVariant=Passthrough  SumFdbkVariant=Disabled  SumVariant=Sum_PI  TsampFilterVariant=InternalTs  TsampNgainVariant=Passthrough  TsampIntegralVariant=Passthrough  ExternalSaturationOutDataTypeStr=Inherit: Same as second input  aMode=0
  Power : Scope
  Power1 : Scope  Commented=on
  Power2 : Scope
  Product : Product
  Product{1..5} (5 alike) : Product  Commented=on
  Product6 : Product
  R_battery : spsSeriesRLCBranchLib/Series RLC Branch  Commented=through  LConnTagsString=__new0  RConnTagsString=__new0  BranchType=R  Resistance=0.1  Inductance=1e-3  SetiL0=off  InitialCurrent=0  Capacitance=1440e-6  Setx0=off  InitialVoltage=80  Measurements=None
  R_battery2 : spsSeriesRLCBranchLib/Series RLC Branch  Commented=through  LConnTagsString=__new0  RConnTagsString=__new0  BranchType=R  Resistance=0.1  Inductance=1e-3  SetiL0=off  InitialCurrent=0  Capacitance=1440e-6  Setx0=off  InitialVoltage=80  Measurements=None
  R_outsideBat : spsSeriesRLCBranchLib/Series RLC Branch  Commented=on  LConnTagsString=__new0  RConnTagsString=__new0  BranchType=R  Resistance=0.1  Inductance=1e-3  SetiL0=off  InitialCurrent=0  Capacitance=1e-6  Setx0=off  InitialVoltage=0  Measurements=None
  R_outsideBat2 : spsSeriesRLCBranchLib/Series RLC Branch  Commented=on  LConnTagsString=__new0  RConnTagsString=__new0  BranchType=R  Resistance=0.1  Inductance=1e-3  SetiL0=off  InitialCurrent=0  Capacitance=1e-6  Setx0=off  InitialVoltage=0  Measurements=None
  Rate Transition{1..4} (4 alike) : RateTransition  Commented=on  OutPortSampleTime=0
  S1_merge2 : Merge  Commented=on  InitialOutput=[0]
  S2_merge2 : Merge  Commented=on  InitialOutput=[0]
  S3_merge2 : Merge  Commented=on  InitialOutput=[0]
  S4_merge2 : Merge  Commented=on  InitialOutput=[0]
  SOC : Scope
  SOC2 : Scope
  Saturation : Saturate  UpperLimit=10  LowerLimit=-10
  Saturation1 : Saturate  UpperLimit=10  LowerLimit=-10  LinearizeAsGain=off
  Saturation2 : Saturate  Commented=on  UpperLimit=10  LowerLimit=-10
  Saturation3 : Saturate  Commented=on  UpperLimit=10  LowerLimit=-10  LinearizeAsGain=off
  Saturation4 : Saturate  Commented=on  UpperLimit=10  LowerLimit=-10
  Saturation5 : Saturate  Commented=on  UpperLimit=10  LowerLimit=-10
  Saturation6 : Saturate  UpperLimit=10  LowerLimit=-10
  Saturation7 : Saturate  UpperLimit=10  LowerLimit=-10  LinearizeAsGain=off
  Scope : Scope  NumInputPorts=3
  Scope1 : Scope  NumInputPorts=3
  Scope2 : Scope  NumInputPorts=3
  Scope3 : Scope  NumInputPorts=2
  Scope4 : Scope
  Scope5 : Scope
  Scope6 : Scope
  Step1 : Step  Commented=on  Time=0.5  Before=88  After=93  SampleTime=0
  Step2 : Step  Commented=on  Time=0.3  Before=5  After=5  SampleTime=0
  Step4 : Step  Commented=on  Time=0.3  Before=1  SampleTime=0
  Step5 : Step  Commented=on  Time=0.3  Before=29  After=5  SampleTime=0
  Step7 : Step  Commented=on  Time=0.5  Before=88  After=93  SampleTime=0
  Step8 : Step  Commented=on  Time=0.3  Before=1  SampleTime=0
  Sum : Sum  Inputs=|+-
  Sum{1..6} (6 alike) : Sum  Commented=on  Inputs=|+-
  Sum10 : Sum  Inputs=|+-
  Sum7 : Sum  Inputs=|++-
  Sum8 : Sum  Inputs=|+-
  Sum9 : Sum  Inputs=|++-
  Switch : Switch  Commented=on  Criteria=u2 > Threshold  SaturateOnIntegerOverflow=off  InputSameDT=off
  Terminator{,1..3,10..13} (8 alike) : Terminator
  Terminator14 : Terminator  Commented=on
  Terminator5 : Terminator  Commented=on
  To Workspace1 : ToWorkspace  Commented=on  VariableName=V_bus_if_input  SaveFormat=Timeseries  SampleTime=-1
  To Workspace2 : ToWorkspace  Commented=on  VariableName=V_bus_if_input1  SaveFormat=Timeseries  SampleTime=-1
  To Workspace3 : ToWorkspace  Commented=on  VariableName=V_battery_if_input1  SaveFormat=Timeseries  SampleTime=-1
  To Workspace4 : ToWorkspace  Commented=on  VariableName=V_battery_if_input  SaveFormat=Timeseries  SampleTime=-1
  Triangle Generator{1..4} (4 alike) : spsTriangleGeneratorLib/Triangle Generator  Commented=on  Freq=wave_freq  Phase=0  Ts=0
  VE{,1..2,6..8} (6 alike) : spsVoltageMeasurementLib/Voltage Measurement  PhasorSimulation=off  OutputType=Complex  PSBequivalent=0
  "V_battery " : Scope
  V_battery 2 : Scope
  V_battery_actual : Scope
  V_battery_actual2 : Scope
  V_bus : Scope
  V_bus2 : Scope
  Vdc 1 : Scope  NumInputPorts=4
  Vdc 3 : Scope  NumInputPorts=4
  Vdc 5 : Scope  Commented=on  NumInputPorts=6
  droop coefficient : Gain  Gain=0.016
  droop coefficient1 : Gain  Gain=0.016
  iL_ref : Scope  Commented=on
  iL_ref_merge2 : Merge  Commented=on  InitialOutput=[0]
  mid_L : spsSeriesRLCBranchLib/Series RLC Branch  LConnTagsString=__new0  RConnTagsString=__new0  BranchType=L  Resistance=1.0  Inductance=40e-6  SetiL0=off  InitialCurrent=10  Capacitance=1.0  Setx0=off  InitialVoltage=0  Measurements=None
  mid_L2 : spsSeriesRLCBranchLib/Series RLC Branch  LConnTagsString=__new0  RConnTagsString=__new0  BranchType=L  Resistance=1.0  Inductance=40e-6  SetiL0=off  InitialCurrent=10  Capacitance=1.0  Setx0=off  InitialVoltage=0  Measurements=None
  mid_R : spsSeriesRLCBranchLib/Series RLC Branch  LConnTagsString=__new0  RConnTagsString=__new0  BranchType=R  Resistance=0.004  Inductance=1e-3  SetiL0=off  InitialCurrent=0  Capacitance=1e-3  Setx0=off  InitialVoltage=80  Measurements=None
  mid_R2 : spsSeriesRLCBranchLib/Series RLC Branch  LConnTagsString=__new0  RConnTagsString=__new0  BranchType=R  Resistance=0.004  Inductance=1e-3  SetiL0=off  InitialCurrent=0  Capacitance=1e-3  Setx0=off  InitialVoltage=80  Measurements=None
  mode_selection : Scope  Commented=on
  u1_merge1 : Merge  Commented=on  InitialOutput=[0]
  u2_merge2 : Merge  Commented=on  InitialOutput=[0]
  + : PMIOPort  Tag=PMCPort  Side=Right
  - : PMIOPort  Tag=PMCPort  Port=2  Side=Right
  tag scope: Battery_SOC2=global, Battery_SOC=global
  wires:
  [S1] -> Vdc 1/1  "S1"
  [S2] -> Vdc 1/2  "S2"
  [S3] -> Vdc 1/3  "S3"
  [S4] -> Vdc 1/4  "S4"
  Sum/1 -> PID Controller2/1
  PID Controller2/1 -> [iL_ref]
  [iL_ref] -> MATLAB Function/1(iL_ref)
  [iL] -> MATLAB Function/2(iL)
  [VC_ref] -> MATLAB Function/3(vc_ref)
  [V_dc] -> MATLAB Function/4(vc)
  [V_battery] -> MATLAB Function/5(vin)
  [Ts] -> MATLAB Function/7(Ts)
  [i_dc] -> MATLAB Function/6(i_out)
  [u1] -> Modulation/1(u1)
  [u2] -> Modulation/2(u2)
  Modulation/1(S1) -> [S1]
  Modulation/3(S3) -> [S3]
  Modulation/4(S4) -> [S4]
  Modulation/2(S2) -> [S2]
  [V_battery] -> Discharge+V/1  "Vin"
  Mux/1 -> Discharge+V/2  "iL"
  [iL_ref] -> Mux/2  "iL*"
  [iL] -> Mux/1  "iL"
  [V_dc] -> Mux1/1  "V_bus"
  [VC_ref] -> Mux1/2  "VC_ref"
  Mux1/1 -> Discharge+V/3  "V_out"
  Mux2/1 -> Discharge+V/6  "u1,u2"
  [u1] -> Mux2/1
  [u2] -> Mux2/2
  VE1/1 -> [V_dc], V_bus/1
  MATLAB Function/2(u2) -> Saturation1/1
  MATLAB Function/1(u1) -> Saturation/1
  [i_dc] -> Discharge+V/4  "i_output"
  [i_battery] -> Discharge+V/5  "i_battery"
  [V_dc] -> Product/1  "Vc"
  [i_dc] -> Product/2  "io"
  Product/1 -> Power/1
  [V_dc] -> Sum/2
  From30/1 -> MATLAB Function1/2(iL)
  From55/1 -> MATLAB Function1/4(i_out)
  From36/1 -> MATLAB Function1/1(iL_ref)
  From37/1 -> MATLAB Function1/3(i_out_ref)
  From33/1 -> MATLAB Function1/5(vin)
  MATLAB Function1/1(u1) -> Saturation4/1
  From35/1 -> MATLAB Function1/7(Ts)
  MATLAB Function1/2(u2) -> Saturation5/1
  From38/1 -> Sum1/1
  Sum1/1 -> PID Controller1/1
  From31/1 -> Sum1/2
  PID Controller1/1 -> Goto20/1
  Modulation1/4(S4) -> Goto21/1
  Modulation1/1(S1) -> Goto23/1
  From40/1 -> Modulation1/2(u2)
  Modulation1/2(S2) -> Goto22/1
  Modulation1/3(S3) -> Goto24/1
  From39/1 -> Modulation1/1(u1)
  From52/1 -> MATLAB Function1/6(Vc)
  From62/1 -> Modulation2/2(u2)
  From61/1 -> Modulation2/1(u1)
  Modulation2/3(S3) -> Goto31/1
  Modulation2/4(S4) -> Goto30/1
  Modulation2/1(S1) -> Goto32/1
  Modulation2/2(S2) -> Goto29/1
  From53/1 -> MATLAB Function2/5(vin)
  From74/1 -> Gain2/1
  From59/1 -> MATLAB Function2/6(Vc)
  From58/1 -> Sum2/1
  From57/1 -> MATLAB Function2/3(i_out_ref)
  PID Controller3/1 -> Goto27/1
  Sum2/1 -> PID Controller3/1
  From54/1 -> MATLAB Function2/7(Ts)
  MATLAB Function2/1(u1) -> Goto15/1
  From56/1 -> MATLAB Function2/1(iL_ref)
  MATLAB Function2/2(u2) -> Goto25/1
  From34/1 -> Gain3/1
  Step2/1 -> Goto26/1
  From32/1 -> Gain/1
  Gain/1 -> MATLAB Function2/2(iL)
  Gain2/1 -> Sum2/2
  Gain3/1 -> MATLAB Function2/4(i_out)
  From87/1 -> Mux10/2  "VC_ref"
  From85/1 -> Gain8/1  "iL"
  From83/1 -> Mux10/1  "V_battery"
  Mux11/1 -> Vdc 5/6  "u1,u2"
  From94/1 -> Sum3/2
  From91/1 -> Vdc 5/5  "i_battery"
  From80/1 -> Modulation3/1(u1)
  From84/1 -> Mux9/2  "iL*"
  Mux9/1 -> Vdc 5/2  "iL"
  From90/1 -> Mux11/2
  From86/1 -> Vdc 5/1  "V_bus"
  PID Controller4/1 -> Goto36/1
  From89/1 -> Mux11/1
  From81/1 -> Modulation3/2(u2)
  Mux10/1 -> Vdc 5/3  "V_out"
  From75/1 -> Sum3/1
  Sum3/1 -> PID Controller4/1
  Modulation3/1(S1) -> Goto41/1
  Modulation3/2(S2) -> Goto28/1
  Modulation3/3(S3) -> Goto40/1
  Modulation3/4(S4) -> Goto33/1
  Gain8/1 -> Mux9/1
  From82/1 -> Vdc 5/4  "i_bus"
  From95/1 -> Gain6/1
  From24/1 -> Gain10/1
  From70/1 -> MATLAB Function3/3(vc_ref)
  From76/1 -> MATLAB Function3/5(vin)
  MATLAB Function3/1(u1) -> Goto6/1
  From77/1 -> MATLAB Function3/4(vc)
  MATLAB Function3/2(u2) -> Goto7/1
  From78/1 -> MATLAB Function3/7(Ts)
  Gain6/1 -> MATLAB Function3/6(i_out)
  Gain10/1 -> MATLAB Function3/2(iL)
  Constant20/1 -> Goto37/1
  From79/1 -> MATLAB Function3/1(iL_ref)
  From174/1 -> Sum5/1
  From193/1 -> Sum5/2
  PID Controller6/1 -> Goto91/1
  Sum5/1 -> PID Controller6/1
  Constant10/1 -> Goto90/1
  Mux16/1 -> Discharge/3  "Power"
  Mux17/1 -> Discharge/6  "u1,u2"
  From187/1 -> Mux16/2
  Mux15/1 -> Discharge/2  "iL"
  From180/1 -> Discharge/1  "V_battery"
  From182/1 -> Mux15/1
  From179/1 -> Mux16/1
  From181/1 -> Mux15/2  "iL*"
  From185/1 -> Mux17/1
  From188/1 -> Divide/1
  From189/1 -> Divide/2
  Divide/1 -> Goto96/1
  From171/1 -> MATLAB Function5/1(iL_ref)
  MATLAB Function5/2(u2) -> Goto89/1
  From173/1 -> Modulation5/1(u1)
  From172/1 -> MATLAB Function5/3(i_out_ref)
  From192/1 -> MATLAB Function5/4(i_out)
  Modulation5/1(S1) -> Goto94/1
  MATLAB Function5/1(u1) -> Goto88/1
  From175/1 -> Modulation5/2(u2)
  From169/1 -> MATLAB Function5/5(vin)
  Modulation5/2(S2) -> Goto93/1
  From168/1 -> MATLAB Function5/2(iL)
  From170/1 -> MATLAB Function5/7(Ts)
  Modulation5/4(S4) -> Goto92/1
  Modulation5/3(S3) -> Goto95/1
  From191/1 -> MATLAB Function5/6(Vc)
  From183/1 -> Mux18/1  "V_bus"
  Mux18/1 -> Discharge/4  "V_out"
  From150/1 -> Mux18/2
  From184/1 -> Mux19/1  "i_bus"
  From177/1 -> Mux19/2  "i_ref"
  Mux19/1 -> Discharge/5  "i_out"
  From186/1 -> Mux17/2
  Constant5/1 -> Goto38/1
  Divide1/1 -> Goto46/1
  From101/1 -> Sum4/1
  Constant12/1 -> Goto100/1
  PID Controller5/1 -> Goto39/1
  Product2/1 -> ActualPower1/1, Goto99/1
  From107/1 -> Gain12/1
  From103/1 -> Divide1/1
  From104/1 -> Product2/1, Divide1/2
  Sum4/1 -> PID Controller5/1
  Mux14/1 -> Charge/6  "u1,u2"
  From195/1 -> Mux14/2
  From178/1 -> Mux21/1  "i_bus"
  From110/1 -> Gain15/1  "i_ref"
  From112/1 -> Charge/1  "V_in"
  Mux21/1 -> Charge/5  "i_out"
  From244/1 -> Mux20/2
  From194/1 -> Mux14/1
  Mux12/1 -> Charge/2  "iL"
  From111/1 -> Mux13/1
  Mux13/1 -> Charge/3  "Power"
  Mux20/1 -> Charge/4  "V_battery"
  From196/1 -> Gain7/1
  From113/1 -> Gain14/1  "iL*"
  From198/1 -> Gain11/1
  Gain11/1 -> Sum4/2
  From114/1 -> Mux12/1
  From108/1 -> Mux20/1
  Gain16/1 -> MATLAB Function6/2(iL)
  MATLAB Function6/2(u2) -> Goto102/1
  From200/1 -> MATLAB Function6/7(Ts)
  From202/1 -> MATLAB Function6/3(i_out_ref)
  From190/1 -> Gain16/1
  From201/1 -> MATLAB Function6/1(iL_ref)
  From199/1 -> MATLAB Function6/5(vin)
  From197/1 -> Gain17/1
  MATLAB Function6/1(u1) -> Goto101/1
  From203/1 -> MATLAB Function6/6(Vc)
  Gain17/1 -> MATLAB Function6/4(i_out)
  Modulation6/3(S3) -> Goto103/1
  From93/1 -> Modulation6/2(u2)
  Modulation6/2(S2) -> Goto34/1
  Modulation6/1(S1) -> Goto104/1
  Modulation6/4(S4) -> Goto35/1
  From64/1 -> Modulation6/1(u1)
  Gain12/1 -> Product2/2
  From97/1 -> Product4/1
  Product4/1 -> BusPower/1, Goto97/1
  From63/1 -> Product4/2
  Constant14/1 -> Goto126/1
  From41/1 -> BatteryCurrent1/1
  Product1/1 -> ActualPower2/1, Goto144/1
  From242/1 -> Product1/1
  From243/1 -> Product1/2
  Constant16/1 -> Goto145/1
  Gain7/1 -> Mux13/2
  Gain15/1 -> Mux21/2
  Gain14/1 -> Mux12/2
  Rate Transition3/1 -> If2/3
  From71/1 -> To Workspace3/1, Rate Transition3/1
  If2/3 -> DoNothing1/Action
  From69/1 -> To Workspace2/1, Rate Transition2/1
  Charge/Discharge Mode2/1 -> If2/1
  Rate Transition2/1 -> If2/2
  Discharge Mixed CurrentPower/1(S1) -> Goto47/1
  From65/1 -> Discharge Mixed CurrentPower/4(I_out)
  From66/1 -> Discharge Mixed CurrentPower/5(TimeStep)
  Discharge Mixed CurrentPower/6(i_out_ref_show) -> Goto51/1
  Discharge Mixed CurrentPower/9(Power_ref_show) -> Goto55/1
  Discharge Mixed CurrentPower/8(u2) -> Goto50/1
  From68/1 -> Discharge Mixed CurrentPower/2(iL)
  Triangle Generator1/1 -> Discharge Mixed CurrentPower/8(Triangular_generator)
  Constant7/1 -> Discharge Mixed CurrentPower/7(Power_ref)
  Constant6/1 -> Discharge Mixed CurrentPower/6(i_out_ref)
  Discharge Mixed CurrentPower/7(u1) -> Goto49/1
  Discharge Mixed CurrentPower/4(S4) -> Goto54/1
  Discharge Mixed CurrentPower/3(S3) -> Goto53/1
  From60/1 -> Discharge Mixed CurrentPower/3(V_battery)
  Discharge Mixed CurrentPower/2(S2) -> Goto52/1
  Discharge Mixed CurrentPower/5(iL_ref) -> Goto48/1
  From67/1 -> Discharge Mixed CurrentPower/1(V_bus)
  If2/1 -> Discharge Mixed CurrentPower/Action
  u1_merge1/1 -> Goto61/1
  iL_ref_merge2/1 -> Goto60/1
  u2_merge2/1 -> Goto62/1
  S4_merge2/1 -> Goto58/1
  S1_merge2/1 -> Goto59/1
  S3_merge2/1 -> Goto57/1
  S2_merge2/1 -> Goto56/1
  From115/1 -> S1_merge2/1
  From116/1 -> S2_merge2/1
  From118/1 -> S3_merge2/1
  From119/1 -> S4_merge2/1
  From120/1 -> iL_ref_merge2/1
  From73/1 -> u1_merge1/1
  From109/1 -> u2_merge2/1
  From121/1 -> Charge Mixed CurrentPower/4(I_battery)
  Constant8/1 -> Charge Mixed CurrentPower/6(i_out_ref)
  From125/1 -> Charge Mixed CurrentPower/2(iL)
  Charge Mixed CurrentPower/8(u2) -> Goto67/1
  Charge Mixed CurrentPower/6(i_out_ref_show) -> Goto68/1
  Charge Mixed CurrentPower/3(S3) -> Goto70/1
  Charge Mixed CurrentPower/2(S2) -> Goto69/1
  Triangle Generator2/1 -> Charge Mixed CurrentPower/7(Triangular_generator)
  From124/1 -> Charge Mixed CurrentPower/1(V_bus)
  Charge Mixed CurrentPower/7(u1) -> Goto66/1
  From123/1 -> Charge Mixed CurrentPower/5(TimeStep)
  From122/1 -> Charge Mixed CurrentPower/3(V_battery)
  Charge Mixed CurrentPower/4(S4) -> Goto71/1
  Charge Mixed CurrentPower/5(iL_ref) -> Goto65/1
  If2/2 -> Charge Mixed CurrentPower/Action
  Charge Mixed CurrentPower/1(S1) -> Goto72/1
  Constant9/1 -> Charge Mixed CurrentPower/8(Power_ref)
  From126/1 -> S1_merge2/2
  From127/1 -> S2_merge2/2
  From128/1 -> S3_merge2/2
  From129/1 -> S4_merge2/2
  From130/1 -> iL_ref_merge2/2
  From132/1 -> u1_merge1/2
  From133/1 -> u2_merge2/2
  Charge Mixed CurrentPower/9(Power_ref_show) -> Goto73/1
  Discharge Mixed CurrentPower/10(iL_PD_out) -> Goto74/1
  [V_dc] -> Divide2/1
  [i_dc] -> Divide2/2
  Divide2/1 -> [Bus_load], Outside Load/1
  From92/1 -> Product3/2  "io"
  From45/1 -> Sum6/1
  From88/1 -> Product3/1  "Vc"
  Modulation4/1(S1) -> Goto77/1
  Modulation4/4(S4) -> Goto42/1
  From49/1 -> Modulation4/1(u1)
  From50/1 -> Modulation4/2(u2)
  PID Controller7/1 -> Goto75/1
  Sum6/1 -> PID Controller7/1
  Modulation4/3(S3) -> Goto78/1
  From98/1 -> Sum6/2
  Product3/1 -> Power1/1
  Modulation4/2(S2) -> Goto43/1
  Constant4/1 -> Goto80/1
  Saturation/1 -> [u1]
  Saturation1/1 -> [u2]
  From139/1 -> Charge Mixed CurrentPower1/2(iL)
  From142/1 -> Discharge Const Voltage/5(TimeStep)
  Charge Mixed CurrentPower1/1(S1) -> Goto114/1
  Triangle Generator3/1 -> Discharge Const Voltage/6(Triangular_generator)
  Charge Mixed CurrentPower1/3(S3) -> Goto112/1
  Charge Mixed CurrentPower1/6(u1) -> Goto108/1
  From136/1 -> Charge Mixed CurrentPower1/3(V_battery)
  From146/1 -> To Workspace4/1, Rate Transition4/1
  Charge Mixed CurrentPower1/2(S2) -> Goto111/1
  From72/1 -> Charge Mixed CurrentPower1/6(i_out_ref)
  From145/1 -> To Workspace1/1, Rate Transition1/1
  Rate Transition1/1 -> If1/2
  If1/2 -> Charge Mixed CurrentPower1/Action
  From137/1 -> Charge Mixed CurrentPower1/5(TimeStep)
  Triangle Generator4/1 -> Charge Mixed CurrentPower1/7(Triangular_generator)
  Charge Mixed CurrentPower1/4(S4) -> Goto113/1
  From141/1 -> Discharge Const Voltage/4(I_out)
  Discharge Const Voltage/1(S1) -> Goto82/1
  Discharge Const Voltage/3(S3) -> Goto98/1
  From138/1 -> Charge Mixed CurrentPower1/1(V_bus)
  Charge Mixed CurrentPower1/7(u2) -> Goto109/1
  Discharge Const Voltage/2(S2) -> Goto87/1
  Charge Mixed CurrentPower1/5(iL_ref) -> Goto107/1
  From140/1 -> Discharge Const Voltage/3(V_battery)
  Discharge Const Voltage/5(iL_ref) -> Goto83/1
  Discharge Const Voltage/6(u1) -> Goto84/1
  Discharge Const Voltage/7(u2) -> Goto85/1
  Charge0 /Discharge1 Mode1/1 -> mode_selection/1, If1/1
  From106/1 -> Charge Mixed CurrentPower1/4(I_battery)
  From143/1 -> Discharge Const Voltage/1(V_bus)
  From144/1 -> Discharge Const Voltage/2(iL)
  If1/3 -> DoNothing2/Action
  If1/1 -> Discharge Const Voltage/Action
  Discharge Const Voltage/4(S4) -> Goto105/1
  Rate Transition4/1 -> If1/3
  Constant19/1 -> Goto117/1
  From147/1 -> Discharge Const Voltage/7(V_bus_ref)
  [Bus_load] -> MATLAB Function/8(Bus_load)
  From156/1 -> MATLAB Function7/8(Bus_load)
  MATLAB Function7/1(u1) -> Saturation2/1
  Saturation3/1 -> Goto119/1
  Saturation2/1 -> Goto81/1
  MATLAB Function7/2(u2) -> Saturation3/1
  From154/1 -> MATLAB Function7/4(vc)
  From155/1 -> MATLAB Function7/5(vin)
  From158/1 -> MATLAB Function7/1(iL_ref)
  From152/1 -> MATLAB Function7/2(iL)
  From157/1 -> MATLAB Function7/7(Ts)
  From153/1 -> MATLAB Function7/3(vc_ref)
  From159/1 -> MATLAB Function7/6(i_out)
  Constant11/1 -> Goto120/1
  Switch/1 -> Goto76/1
  From47/1 -> Switch/3
  From48/1 -> Product5/1
  From51/1 -> Product5/2
  Product5/1 -> Switch/1
  From46/1 -> Minus/1
  From44/1 -> Minus/2
  From100/1 -> iL_ref/1  "iL*"
  Minus/1 -> Switch/2
  From99/1 -> Discharge Const Voltage/8(Bus_load)
  From102/1 -> If1/4
  Step5/1 -> Goto19/1
  Saturation4/1 -> Goto17/1
  Saturation5/1 -> Goto18/1
  Constant2/1 -> Goto45/1
  [Ubus_ref] -> Sum7/2
  droop coefficient/1 -> Sum7/3, Scope1/2
  [i_dc] -> Scope1/3, droop coefficient/1
  Sum7/1 -> Scope1/1, [VC_ref]
  [VC_ref] -> Sum/1
  Constant13/1 -> [Ubus_ref]
  Current 1/1 -> Scope/1, [i_dc], Low-Pass Filter (Discrete or Continuous)/1
  [iL_ref2] -> MATLAB Function4/1(iL_ref)
  [iL2] -> MATLAB Function4/2(iL)
  [Ubus_ref] -> Sum9/2
  [u12] -> Modulation7/1(u1)
  [VC_ref2] -> Sum8/1
  [i_dc2] -> Scope2/3, droop coefficient1/1
  [Bus_load2] -> MATLAB Function4/8(Bus_load)
  [u12] -> Mux5/1
  Saturation7/1 -> [u22]
  Mux5/1 -> Discharge+V1/6  "u1,u2"
  droop coefficient1/1 -> Sum9/3, Scope2/2
  [iL2] -> Mux3/1  "iL"
  Modulation7/1(S1) -> [S12]
  [i_dc2] -> Product6/2  "io"
  Mux4/1 -> Discharge+V1/3  "V_out"
  PID Controller8/1 -> [iL_ref2]
  Mux3/1 -> Discharge+V1/2  "iL"
  [V_dc2] -> Product6/1  "Vc"
  [VC_ref2] -> MATLAB Function4/3(vc_ref)
  Modulation7/2(S2) -> [S22]
  Saturation6/1 -> [u12]
  [u22] -> Mux5/2
  [V_battery2] -> Discharge+V1/1  "Vin"
  MATLAB Function4/2(u2) -> Saturation7/1
  [i_battery2] -> Discharge+V1/5  "i_battery"
  Modulation7/4(S4) -> [S42]
  [VC_ref2] -> Mux4/2  "VC_ref"
  [u22] -> Modulation7/2(u2)
  [V_dc2] -> Sum8/2
  Sum9/1 -> Scope2/1, [VC_ref2]
  [iL_ref2] -> Mux3/2  "iL*"
  [V_battery2] -> MATLAB Function4/5(vin)
  [i_dc2] -> Discharge+V1/4  "i_output"
  Product6/1 -> Power2/1
  [Ts2] -> MATLAB Function4/7(Ts)
  Modulation7/3(S3) -> [S32]
  [V_dc2] -> MATLAB Function4/4(vc)
  [i_dc2] -> MATLAB Function4/6(i_out)
  MATLAB Function4/1(u1) -> Saturation6/1
  Sum8/1 -> PID Controller8/1
  [V_dc2] -> Mux4/1  "V_bus"
  Current Measurement/1 -> [iL], InductorCurrent/1
  Bus Selector/1 -> [Battery_SOC], SOC/1  "<SOC (%)>"
  [S4] -> IGBT/Diode4/1
  [S3] -> IGBT/Diode3/1
  "85 volts, 100 Ah LithiumIon battery "/1 -> Bus Selector/1
  Step1/1 -> Controlled Voltage Source/1
  VE2/1 -> [V_battery_actual], V_battery_actual/1
  Step4/1 -> Ideal Switch3/1
  Divide3/1 -> Battery Load/1
  IGBT/Diode1/1 -> Terminator/1
  Constant1/1 -> [Ts]
  VE/1 -> [V_battery], "V_battery "/1
  IGBT/Diode4/1 -> Terminator2/1
  IGBT/Diode2/1 -> Terminator1/1
  IL6/1 -> Scope4/1, [i_battery]
  [S1] -> IGBT/Diode1/1  "S1"
  Ideal Switch3/1 -> Terminator5/1
  [S2] -> IGBT/Diode2/1
  [i_battery] -> Divide3/2
  IGBT/Diode3/1 -> Terminator3/1
  [V_battery_actual] -> Divide3/1
  Ideal Switch2/1 -> Terminator14/1
  IGBT/Diode11/1 -> Terminator13/1
  [i_battery2] -> Divide7/2
  [S22] -> IGBT/Diode10/1
  Constant17/1 -> [Ts2]
  VE8/1 -> [V_battery_actual2], V_battery_actual2/1
  [S12] -> IGBT/Diode9/1  "S1"
  Bus Selector2/1 -> [Battery_SOC2], SOC2/1  "<SOC (%)>"
  Step8/1 -> Ideal Switch2/1
  Current Measurement2/1 -> [iL2], InductorCurrent2/1
  [S42] -> IGBT/Diode12/1
  [S32] -> IGBT/Diode11/1
  "85 volts, 100 Ah LithiumIon battery 2"/1 -> Bus Selector2/1
  [S12] -> Vdc 3/1  "S1"
  Step7/1 -> Controlled Voltage Source2/1
  IGBT/Diode9/1 -> Terminator10/1
  [i_dc2] -> Divide6/2
  [S42] -> Vdc 3/4  "S4"
  [V_battery_actual2] -> Divide7/1
  IGBT/Diode10/1 -> Terminator11/1
  IGBT/Diode12/1 -> Terminator12/1
  Divide6/1 -> Outside Load2/1, [Bus_load2]
  VE6/1 -> [V_battery2], V_battery 2/1
  VE7/1 -> [V_dc2], V_bus2/1
  Current 2/1 -> Scope5/1, Scope/2, [i_dc2], Low-Pass Filter (Discrete or Continuous)1/1
  Divide7/1 -> Battery Load2/1
  IL2/1 -> Scope6/1, [i_battery2]
  [V_dc2] -> Divide6/1
  [S32] -> Vdc 3/3  "S3"
  [S22] -> Vdc 3/2  "S2"
  Current total/1 -> Scope/3, [i_total]
  Low-Pass Filter (Discrete or Continuous)/1 -> Goto131/1
  Low-Pass Filter (Discrete or Continuous)1/1 -> Goto138/1
  [delta_Uref] -> Sum7/1
  [delta_Uref] -> Sum9/1
  Sum10/1 -> PID Controller/1, Scope3/2
  [Ubus_ref] -> Sum10/1
  [VC] -> Sum10/2, Scope3/1
  PID Controller/1 -> [delta_Uref]
  connections:
  C2/LConn1 -- VE1/LConn1 -- DM_inductor2/LConn1 -- IGBT/Diode3/LConn1
  DM_inductor2/RConn1 -- Current 1/LConn1
  DM_inductor1/RConn1 -- C1/LConn1 -- IGBT/Diode1/LConn1 -- VE/LConn1
  R_battery/LConn1 -- "85 volts, 100 Ah LithiumIon battery "/LConn2 -- VE2/LConn2
  IGBT/Diode2/LConn1 -- IGBT/Diode1/RConn1 -- mid_R/RConn1
  IGBT/Diode3/RConn1 -- IGBT/Diode4/LConn1 -- Current Measurement/RConn1
  mid_R/LConn1 -- mid_L/LConn1
  Controlled Voltage Source/LConn1 -- R_outsideBat/LConn1
  mid_L/RConn1 -- Current Measurement/LConn1
  Ideal Switch3/LConn1 -- Controlled Voltage Source/RConn1
  IL6/RConn1 -- DM_inductor1/LConn1
  Current 1/RConn1 -- Current 2/RConn1 -- Current total/LConn1
  C6/RConn1 -- R_outsideBat2/RConn1 -- R_battery2/RConn1 -- C5/RConn1 -- VE6/LConn2 -- IGBT/Diode10/RConn1 -- IGBT/Diode12/RConn1 -- C2/RConn1 -- VE1/LConn2 -- IGBT/Diode4/RConn1 -- R_outsideBat/RConn1 -- R_battery/RConn1 -- C1/RConn1 -- VE/LConn2 -- IGBT/Diode2/RConn1 -- -/RConn1 -- VE7/LConn2
  IL6/LConn1 -- "85 volts, 100 Ah LithiumIon battery "/LConn1 -- VE2/LConn1 -- Ideal Switch3/RConn1
  mid_R2/RConn1 -- IGBT/Diode10/LConn1 -- IGBT/Diode9/RConn1
  Ideal Switch2/RConn1 -- IL2/LConn1 -- "85 volts, 100 Ah LithiumIon battery 2"/LConn1 -- VE8/LConn1
  Current Measurement2/RConn1 -- IGBT/Diode11/RConn1 -- IGBT/Diode12/LConn1
  VE6/LConn1 -- IGBT/Diode9/LConn1 -- C5/LConn1 -- DM_inductor5/RConn1
  IGBT/Diode11/LConn1 -- C6/LConn1 -- VE7/LConn1 -- DM_inductor6/LConn1
  VE8/LConn2 -- R_battery2/LConn1 -- "85 volts, 100 Ah LithiumIon battery 2"/LConn2
  mid_R2/LConn1 -- mid_L2/LConn1
  Controlled Voltage Source2/LConn1 -- R_outsideBat2/LConn1
  IL2/RConn1 -- DM_inductor5/LConn1
  Ideal Switch2/LConn1 -- Controlled Voltage Source2/RConn1
  mid_L2/RConn1 -- Current Measurement2/LConn1
  DM_inductor6/RConn1 -- Current 2/LConn1
  Current total/RConn1 -- +/RConn1
